simulink model "adc1_sub2_masked_checkboxes2"  (R2018b)
settings: Solver=ode45  StartTime=0.0  StopTime=10e-05  RelTol=1e-3  EnableMultiTasking=on
libraries: dsparch4 x2
settings Model: Creator=bbhattac  LastModifiedBy=khung
settings DataIOCC: LimitDataPoints=on  SaveFormat=Array
settings OptimizationCC: ExpressionDepthLimit=2147483647  LifeSpan=inf
settings DebuggingCC: UnderspecifiedInitializationDetection=Classic  MergeDetectMultiDrivingBlocksExec=none  SolverPrmCheckMsg=warning  ParameterPrecisionLossMsg=none  FcnCallInpInsideContextMsg=warning  StateNameClashWarn=warning  SFUnexpectedBacktrackingDiag=warning  SFNoUnconditionalDefaultTransitionDiag=warning  SFExecutionAtInitializationDiag=none
settings HardwareCC: ProdBitPerPointer=32  ProdBitPerSizeT=32  ProdBitPerPtrDiffT=32  ProdLargestAtomicFloat=None  ProdIntDivRoundTo=Undefined  ProdEndianess=Unspecified  ProdWordSize=32  ProdHWDeviceType=32-bit Generic
settings ModelReferenceCC: PropagateSignalLabelsOutOfModel=off
settings SFSimCC: SimUseLocalCustomCode=off
settings RTWCC: RTWUseLocalCustomCode=off
settings CodeAppCC: StateflowObjectComments=on
settings GRTTargetCC: TargetLangStandard=C89/C90 (ANSI)  GeneratePreprocessorConditionals=Disable all  CombineOutputUpdateFcns=off  GRTInterface=on
settings ConfigComp: CovMetricSettings=dw  CovHtmlReporting=on  CovSaveCumulativeToWorkspaceVar=on  CovSaveSingleToWorkspaceVar=on  CovExternalEMLEnable=off

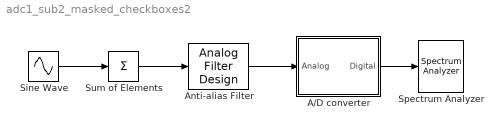
== system adc1_sub2_masked_checkboxes2 ==
  A/D converter : Subsystem  mask(A/D converter){jitter_on=on, minDelay=1.0e-09, maxDelay=15.0e-09, nonlinearity_on=on, nonlingain=0.2, quantization_on=on, nbits=8}
      mask prompts: jitter_on "Enable jitter"; minDelay "Minimum aperture delay"; maxDelay "Maximum aperture delay"; nonlinearity_on "Enable nonlinearity"; nonlingain "Nonlinear gain"; quantization_on "Enable quantization and saturation"; nbits "No. of quantization bits"
      mask help: Simulates typical ADC impairments. Mask parameters control the degree of impairment simulated by the block.
      mask Help:
      | Minimum aperture delay and Maximum aperture delay: These control the aperture jitter for the ADC.
      | 
      | Nonlinear gain: This parameter controls the amount of nonlinear distortion in the ADC transfer function.
      | 
      | No. of quantization bits: Specifies the number of quantization bits for the ADC.
      mask Callback jitter_on:
      | en = get_param(gcb,'MaskEnables');
      | 
      | if strcmp(get_param(gcb,'jitter_on'),'on')
      |         en{2} = 'on';
      |         en{3} = 'on';
      | else
      |         en{2} = 'off';
      |         en{3} = 'off';
      | end
      | set_param(gcb,'MaskEnables',en)
      mask Callback nonlinearity_on:
      | en = get_param(gcb,'MaskEnables');
      | 
      | if strcmp(get_param(gcb,'nonlinearity_on'),'on')
      |         en{5} = 'on';
      | else
      |         en{5} = 'off';
      | end
      | set_param(gcb,'MaskEnables',en)
      mask Callback quantization_on:
      | en = get_param(gcb,'MaskEnables');
      | 
      | if strcmp(get_param(gcb,'quantization_on'),'on')
      |         en{7} = 'on';
      | else
      |         en{7} = 'off';
      | end
      | set_param(gcb,'MaskEnables',en)
      mask DialogControl ParameterTabVar0 Prompt: Jitter
      mask DialogControl ParameterTabVar01 Prompt: Nonlinearity
      mask DialogControl ParameterTabVar012 Prompt: Quantization and Saturation
      mask Display:
      | plot([0,1,1,2,2,3,3,4,4],[0,0,1,1,2,2,3,3,4]);
      | plot([0,4],[2,2]);
      | plot([2,2],[0,4]);
      | % Note that you don't need to specify 'hold on'
      | % to keep plotting on the same axis for the icon.
      | text(0.3,3,'ADC');
  Anti-alias Filter : dsparch4/Analog Filter Design  method=Butterworth  filttype=Lowpass  N=8  Wlo=2*pi*50e+06  Whi=80  Rp=2  Rs=40
  Sine Wave : Sin  Amplitude=0.25  Frequency=2*pi*[20 22]*1e6  SampleTime=0
  Spectrum Analyzer : SpectrumAnalyzer
  Sum of Elements : Sum  Inputs=+
  wires:
  Sine Wave/1 -> Sum of Elements/1
  Sum of Elements/1 -> Anti-alias Filter/1
  Anti-alias Filter/1 -> A/D converter/1(Analog)
  A/D converter/1(Digital) -> Spectrum Analyzer/1

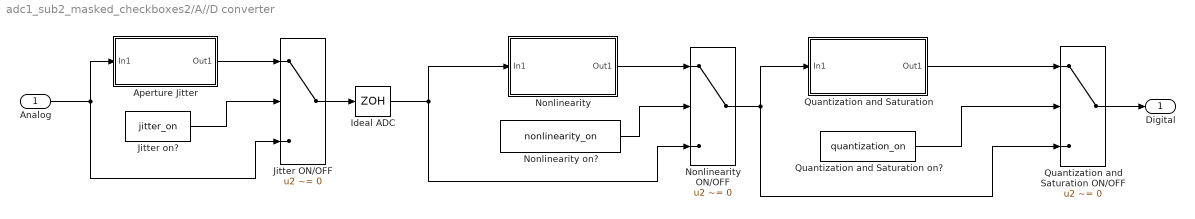
== system adc1_sub2_masked_checkboxes2/A//D converter ==
  Analog : Inport
  Aperture Jitter : Subsystem
  Ideal ADC : ZeroOrderHold  SampleTime=1/100e6
  Jitter ON/OFF : Switch  Criteria=u2 ~= 0
  Jitter on? : Constant  Value=jitter_on
  Nonlinearity : Subsystem
  Nonlinearity ON/OFF : Switch  Criteria=u2 ~= 0
  Nonlinearity on? : Constant  Value=nonlinearity_on
  Quantization and Saturation : Subsystem
  Quantization and Saturation ON/OFF : Switch  Criteria=u2 ~= 0
  Quantization and Saturation on? : Constant  Value=quantization_on
  Digital : Outport
  wires:
  Quantization and Saturation on?/1 -> Quantization and Saturation ON/OFF/2
  Nonlinearity on?/1 -> Nonlinearity ON/OFF/2
  Jitter on?/1 -> Jitter ON/OFF/2
  Aperture Jitter/1(Out1) -> Jitter ON/OFF/1
  Quantization and Saturation ON/OFF/1 -> Digital/1
  Nonlinearity/1(Out1) -> Nonlinearity ON/OFF/1
  Nonlinearity ON/OFF/1 -> Quantization and Saturation/1(In1), Quantization and Saturation ON/OFF/3
  Quantization and Saturation/1(Out1) -> Quantization and Saturation ON/OFF/1
  Ideal ADC/1 -> Nonlinearity/1(In1), Nonlinearity ON/OFF/3
  Jitter ON/OFF/1 -> Ideal ADC/1
  Analog/1 -> Jitter ON/OFF/3, Aperture Jitter/1(In1)

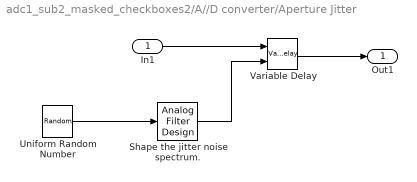
== system adc1_sub2_masked_checkboxes2/A//D converter/Aperture Jitter ==
  In1 : Inport
  "Shape the jitter noise spectrum. " : dsparch4/Analog Filter Design  method=Butterworth  filttype=Lowpass  N=3  Wlo=2*pi*20e6  Whi=80  Rp=2  Rs=40
  Uniform Random Number : UniformRandomNumber  Minimum=minDelay  Maximum=maxDelay  Seed=1234  SampleTime=0
  Variable Delay : VariableTransportDelay  MaximumDelay=1.1*maxDelay  ZeroDelay=on  TransDelayFeedthrough=on
  Out1 : Outport
  wires:
  Variable Delay/1 -> Out1/1
  In1/1 -> Variable Delay/1
  "Shape the jitter noise spectrum. "/1 -> Variable Delay/2
  Uniform Random Number/1 -> "Shape the jitter noise spectrum. "/1

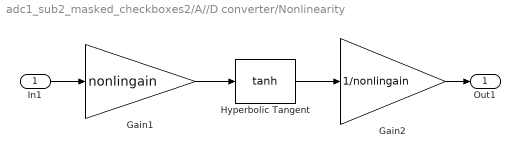
== system adc1_sub2_masked_checkboxes2/A//D converter/Nonlinearity ==
  In1 : Inport
  Gain1 : Gain  Gain=nonlingain  SaturateOnIntegerOverflow=on  OutDataTypeStr=Inherit: Same as input  ParamDataTypeStr=Inherit: Same as input
  Gain2 : Gain  Gain=1/nonlingain  SaturateOnIntegerOverflow=on  OutDataTypeStr=Inherit: Same as input  ParamDataTypeStr=Inherit: Same as input
  Hyperbolic Tangent : Trigonometry  Operator=tanh
  Out1 : Outport
  wires:
  Gain2/1 -> Out1/1
  In1/1 -> Gain1/1
  Gain1/1 -> Hyperbolic Tangent/1
  Hyperbolic Tangent/1 -> Gain2/1

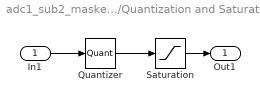
== system adc1_sub2_masked_checkboxes2/A//D converter/Quantization and Saturation ==
  In1 : Inport
  Quantizer : Quantizer  QuantizationInterval=2^-nbits
  Saturation : Saturate
  Out1 : Outport
  wires:
  Saturation/1 -> Out1/1
  In1/1 -> Quantizer/1
  Quantizer/1 -> Saturation/1
